simulink model "Exer1"  (R2014b)
settings: Solver=ode45  StartTime=0.0  StopTime=2  RelTol=1e-3
settings Model: Creator=Charlie  LastModifiedBy=Charlie

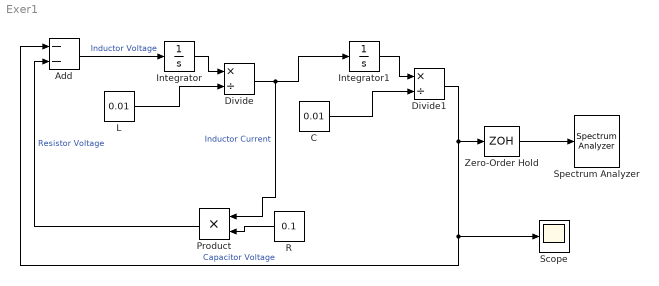
== system Exer1 ==
  Add : Sum  Inputs=--
  C : Constant  Value=0.01
  Divide : Product  Inputs=*/
  Divide1 : Product  Inputs=*/
  Integrator : Integrator  InitialCondition=0.1
  Integrator1 : Integrator  InitialCondition=0.1
  L : Constant  Value=0.01
  Product : Product
  R : Constant  Value=0.1
  Scope : Scope
      settings: TimeRange=9.998000000000645e-07  YMin=12.4355  YMax=12.4362
  Spectrum Analyzer : SpectrumAnalyzer
  Zero-Order Hold : ZeroOrderHold  SampleTime=2e-4
  wires:
  Add/1 -> Integrator/1  "Inductor Voltage"
  Integrator/1 -> Divide/1
  L/1 -> Divide/2
  Divide/1 -> Product/1, Integrator1/1  "Inductor Current"
  Integrator1/1 -> Divide1/1
  C/1 -> Divide1/2
  Divide1/1 -> Zero-Order Hold/1, Scope/1, Add/1  "Capacitor Voltage"
  R/1 -> Product/2
  Product/1 -> Add/2  "Resistor Voltage"
  Zero-Order Hold/1 -> Spectrum Analyzer/1
